simulink model "open_Buck_Boost"  (R2020b)
settings: Solver=VariableStepAuto  StartTime=0.0  StopTime=0.05  RelTol=1e-3
values from neighbouring files (symbols this model uses):
  C = 1e-5    (= 1e-05)    [main_accurate_Runknown.m]
  L = 1.2e-4    (= 0.00012)    [main_accurate_Runknown.m]
  R = 50    [main_accurate_Runknown.m]
  T = 1e-7    (= 1e-07)    [main_accurate_Runknown.m]
  Vin = 20    [main_accurate_Runknown.m]
libraries: powerlib x10, powerlib_meascontrol x1
settings Model: Creator=Asus  LastModifiedBy=Asus

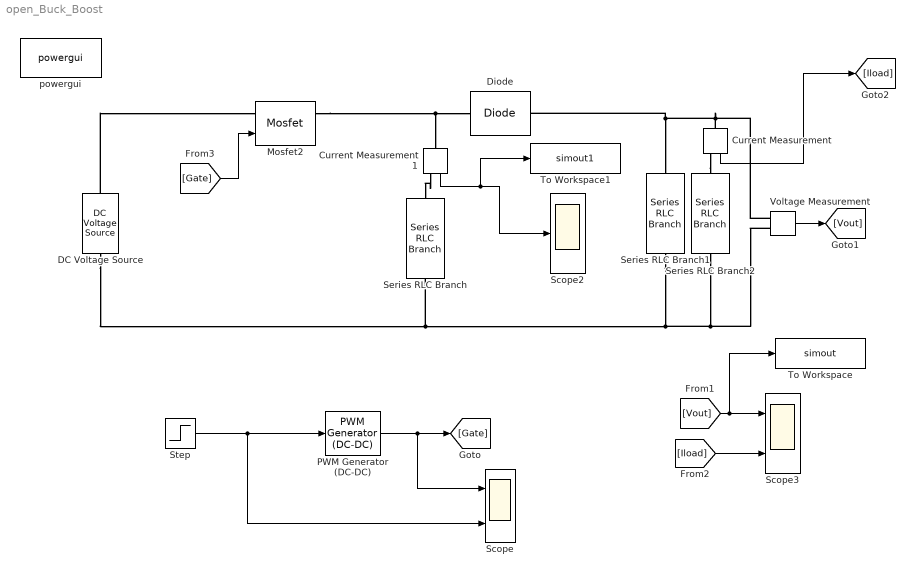
== system open_Buck_Boost ==
  Current Measurement : powerlib/Measurements/Current Measurement  PhasorSimulation=off  OutputType=Complex  PSBequivalent=0
  Current Measurement1 : powerlib/Measurements/Current Measurement  PhasorSimulation=off  OutputType=Complex  PSBequivalent=0
  DC Voltage Source : powerlib/Electrical Sources/DC Voltage Source  Amplitude=Vin  Measurements=None
  Diode : powerlib/Power Electronics/Diode  Ron=0  Lon=0  Vf=0  IC=0  UseSnubber=0  Rs=5e3  Cs=250e-9  Measurements=off
  Mosfet2 : powerlib/Power Electronics/Mosfet  Ron=0  Lon=0  Rd=0  Vfd=0  IC=0  Rs=1e5  Cs=inf  Measurements=on
  PWM Generator (DC-DC) : powerlib_meascontrol/Pulse & Signal Generators/PWM Generator (DC-DC)  Fsw=fre  Ts=0
  Scope : Scope  NumInputPorts=2
  Scope2 : Scope
  Scope3 : Scope  NumInputPorts=2
  Series RLC Branch : powerlib/Elements/Series RLC Branch  LConnTagsString=__new0  RConnTagsString=__new0  BranchType=L  Resistance=1  Inductance=L  SetiL0=off  InitialCurrent=0  Capacitance=1e-6  Setx0=off  InitialVoltage=0  Measurements=None
  Series RLC Branch1 : powerlib/Elements/Series RLC Branch  LConnTagsString=__new0  RConnTagsString=__new0  BranchType=C  Resistance=1  Inductance=1e-3  SetiL0=off  InitialCurrent=0  Capacitance=C  Setx0=off  InitialVoltage=0  Measurements=None
  Series RLC Branch2 : powerlib/Elements/Series RLC Branch  LConnTagsString=__new0  RConnTagsString=__new0  BranchType=R  Resistance=R  Inductance=1e-3  SetiL0=off  InitialCurrent=0  Capacitance=200e-6  Setx0=off  InitialVoltage=0  Measurements=None
  Step : Step  Time=0  After=0.5  SampleTime=0
  To Workspace : ToWorkspace  VariableName=simout  SampleTime=T
      settings: Save2DSignal=2-D array (concatenate along first dimension)
  To Workspace1 : ToWorkspace  VariableName=simout1  SampleTime=T
      settings: Save2DSignal=2-D array (concatenate along first dimension)
  Voltage Measurement : powerlib/Measurements/Voltage Measurement  PhasorSimulation=off  OutputType=Complex  PSBequivalent=0
  powergui : powerlib/powergui  Priority=1  SimulationMode=Continuous  SampleTime=1e-6  frequency=60  Iterations=50  frequencyindice=0  Pbase=100e6  ErrMax=1e-4  UnitsV=kV  UnitsW=MW  buscounter=0  FunctionMessages=off  echomessages=off  EnableUseOfTLC=off  CurrentSourceSwitches=off  DisableSnubberDevices=off  DisableRonSwitches=off  DisableVfSwitches=off  DisplayEquations=off  AutomaticDiscreteSolvers=off  SolverType=Tustin/Backward Euler (TBE)  Interpol=off  ExternalGateDelay=off  methode=off  Ts=100  x0status=blocks  SPID=on  SwTol=0  HookPort=off  NonlinearTolerance=1e-4  nMaxIteration=100  ContinueOnMaxIteration=off  RestoreLinks=warning  ResistiveCurrentMeasurement=off  Frange=[0:2:500]  Ylog=off  Xlog=on  ShowGrid=off  save=off  variable=ZData  structure=0  ZoomFFT=off  StartTime=0.0  cycles=1  DisplayStyle=1  fundamental=60  FreqAxis=off  MaxFrequency=1000  frequencyindicesteady=1  RmsSteady=1  display=off
  wires:
  Step/1 -> Scope/2, PWM Generator (DC-DC)/1
  [Iload] -> Scope3/2
  Current Measurement/1 -> [Iload]
  [Vout] -> To Workspace/1, Scope3/1
  PWM Generator (DC-DC)/1 -> Scope/1, [Gate]
  Voltage Measurement/1 -> [Vout]
  [Gate] -> Mosfet2/1
  Current Measurement1/1 -> To Workspace1/1, Scope2/1
  connections:
  Series RLC Branch2/RConn1 -- DC Voltage Source/LConn1 -- Series RLC Branch/RConn1 -- Series RLC Branch1/RConn1 -- Voltage Measurement/LConn2
  Mosfet2/RConn1 -- Diode/RConn1 -- Current Measurement1/LConn1
  Current Measurement/RConn1 -- Series RLC Branch2/LConn1
  Current Measurement/LConn1 -- Voltage Measurement/LConn1 -- Diode/LConn1 -- Series RLC Branch1/LConn1
  DC Voltage Source/RConn1 -- Mosfet2/LConn1
  Current Measurement1/RConn1 -- Series RLC Branch/LConn1
